simulink model "montage"  (Simulink 7.5)
settings: Solver=ode45  StartTime=0.0  StopTime=Tsim  RelTol=1e-3
values from neighbouring files (symbols this model uses):
  Fsin = (25)*2*pi    (= 157.079632679)    [fft_script.m]    (also in script.m)
  Te = 1/Fe    (= 3.125e-06)    [Bode_partie1.m]    (also in fft_script.m = 0.03125; script.m = 0.03125; script1.m; script2.m)
settings Model: Creator=vendome  LastModifiedBy=Yann
settings DebuggingCC: FcnCallInpInsideContextMsg=Enable All
settings GRTTargetCC: CombineOutputUpdateFcns=on

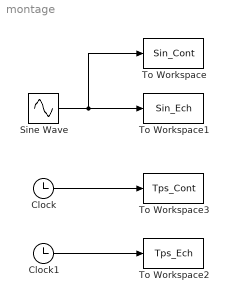
== system montage ==
  Clock : Clock
      settings: Decimation=10
  Clock1 : Clock
      settings: Decimation=10
  Sine Wave : Sin  Amplitude=1  Bias=0  Frequency=Fsin  Phase=0  Samples=10  SampleTime=0  Offset=0
  To Workspace : ToWorkspace  VariableName=Sin_Cont  SampleTime=Te/100  SaveFormat=Array
  To Workspace1 : ToWorkspace  VariableName=Sin_Ech  SampleTime=Te  SaveFormat=Array
  To Workspace2 : ToWorkspace  VariableName=Tps_Ech  SampleTime=Te  SaveFormat=Array
  To Workspace3 : ToWorkspace  VariableName=Tps_Cont  SampleTime=Te/100  SaveFormat=Array
  wires:
  Sine Wave/1 -> To Workspace1/1, To Workspace/1
  Clock/1 -> To Workspace3/1
  Clock1/1 -> To Workspace2/1
